simulink model "StateFlow_2"  (R2018a)
settings: Solver=VariableStepDiscrete  StartTime=0.0  StopTime=10  MaxStep=0.01  RelTol=1e-3
settings Model: SnapshotBufferSize=1000  Creator=Choaib ELMADI  LastModifiedBy=Choaib ELMADI

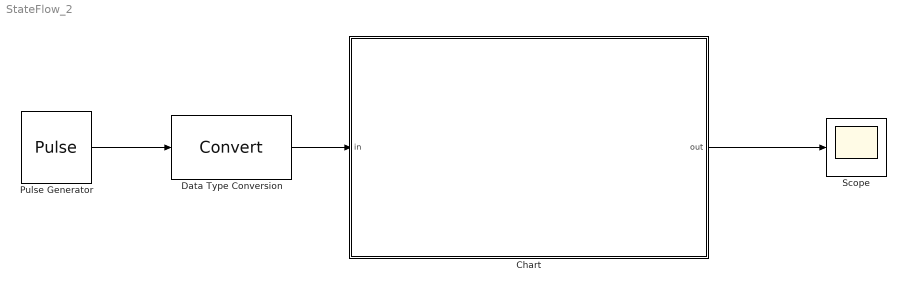
== system StateFlow_2 ==
  Chart : Stateflow chart  TreatAsAtomicUnit=on
  Data Type Conversion : DataTypeConversion
  Pulse Generator : DiscretePulseGenerator  PulseType=Time based  Period=0.1  PulseWidth=50
  Scope : Scope
  wires:
  Pulse Generator/1 -> Data Type Conversion/1
  Data Type Conversion/1 -> Chart/1(in)
  Chart/1(out) -> Scope/1

== stateflow chart StateFlow_2/Chart ==
  state ON_STATE
    en:
    out=1
    du:
    out=2
    ex:
    out=4
    on every(3, tick):
    out=3
  state OFF_STATE
    en:
    out=5
    du:
    out=6
    ex:
    out=8
    on every(3, tick):
    out=7
  (default) -> ON_STATE
  ON_STATE -> OFF_STATE : [in==0]
  OFF_STATE -> ON_STATE : [in==1]
  data: in input double; out output double
